simulink model "Copy_5_of_baseModel"  (R2019a)
settings: Solver=ode1  StartTime=0.0  StopTime=2.5  FixedStep=Ts_Power  RelTol=1e-3
PostLoadFcn:
  | %% Init for wind PnO models - global system parameters
  | OVERRIDE_SSN_MEMORY_LIMIT=1;
  | Ts=50e-6;
  | % Ts=50e-10;
  | Ts_Power=Ts;
  | Ts_Control=2*Ts;
  | freq = 50;
  | Fnom=freq;
  | Vac=400e3;
InitFcn:
  | %% Init for wind PnO models - global system parameters
  | OVERRIDE_SSN_MEMORY_LIMIT=1;
  | Ts=50e-6;
  | % Ts=50e-10;
  | Ts_Power=Ts;
  | Ts_Control=2*Ts;
  | freq = 50;
  | Fnom=freq;
  | Vac=225e3;
values from neighbouring files (symbols this model uses):
  ohl_posCap = (0.01e-006)*12    (= 1.2e-07)    [variable.m]
  ohl_posInd = (1.15e-3)/12    (= 9.58333333333e-05)    [variable.m]
  ohl_posR = 0.069/12    (= 0.00575)    [variable.m]
  ohl_zeroCap = (0.004e-006)*12    (= 4.8e-08)    [variable.m]
  ohl_zeroInd = (2.86e-3)/12    (= 0.000238333333333)    [variable.m]
  ohl_zeroR = 0.1725/12    (= 0.014375)    [variable.m]
  sub_posCap = sub_posCap*6    (= 9.6e-07)    [variable.m]
  sub_posInd = sub_posInd/6    (= 0.000233333333333)    [variable.m]
  sub_posR = sub_posR/6    (= 0.006)    [variable.m]
  sub_zeroCap = sub_zeroCap*6    (= 3.84e-07)    [variable.m]
  sub_zeroInd = sub_zeroInd/6    (= 0.000583333333333)    [variable.m]
  sub_zeroR = sub_zeroR/6    (= 0.015)    [variable.m]
  transfo_L1 = 0.05999374    [variable.m]
  transfo_L2 = 0.05999374    [variable.m]
  transfo_R1 = 0.000866667    [variable.m]
  transfo_R2 = 0.00086667    [variable.m]
undefined symbols (not defined in the file or in its folder): D1, D11, Delta, den, DiscIntNeverNeededParam, dx, find_system, gcbh, num, out_Buses, out_WindFarms, sps_rtmsupport
libraries: powerlib x200, simulink x96, powerlib_meascontrol x96, elements x52, eeSinusoidalMeasurement x51, simulink_extras x42, spsVIMeasurementModel x36, eePowerMeasurement x16
(part 19 of 24)

== system Copy_5_of_baseModel/SM_WT1/Overcurrent Element 2/Overcurrent Relay Scheme/Analog filtering, signal conditioning/CURRENTS ==
  Iabc : Inport
  Abs{,1..3} (4 alike) : Abs
  Add : Sum  Inputs=+++
  Complex : MagnitudeAngleToComplex
  Complex1 : MagnitudeAngleToComplex
  Complex2 : MagnitudeAngleToComplex
  Constant : Constant  Value=pi/180
  DAB - current A : Subsystem  AncestorBlock=elements/DAB  mask(Data Adquisition Board){filter=off, approx=Butterworth, order=2, numerator=[], denominator=[], freq=fCut, resdis=off, vertres=16, xmax=CurrentRange, winsize=WindowSize, G=1.0, fs=fSampling}
      mask prompts: filter "Disable Analog Filter"; approx "Filter approximation"; numerator "Free expression filter: numerator(descending order of s)"; denominator "Free expression filter: denominator:"; freq "Cut-off frequency"; resdis "Disable Vertical Resolution"; vertres "Vertical Resolution: No. of bits"; xmax "Vertical Resolution: signal range"; winsize "Window size"; G "Gain"; fs "Sampling frequency"
      mask help: Performs analog filtering, signal conditioning and sampling. A single signal is the input, a buffer with the signal samples is the output. The options include analog filter enable/disable switch, type, order and cut-off frequency of the analog filter, conditioning gain, sampling frequency, number of bits, the length of the buffer.
      mask init:
      | dab1
      mask Help: web(['file:///' which('dabdoc2.html')]);
      mask TypeOptions approx: Bessel | Tschebyscheff | Butterworth | free expression
      mask TypeOptions order: 2 | 3 | 4
      mask TypeOptions vertres: 8 | 12 | 16
      mask Display: disp('DAB')
  DAB - current B : Subsystem  AncestorBlock=elements/DAB  mask(Data Adquisition Board){filter=off, approx=Butterworth, order=2, numerator=[], denominator=[], freq=fCut, resdis=off, vertres=16, xmax=CurrentRange, winsize=WindowSize, G=1.0, fs=fSampling}
      mask prompts: filter "Disable Analog Filter"; approx "Filter approximation"; numerator "Free expression filter: numerator(descending order of s)"; denominator "Free expression filter: denominator:"; freq "Cut-off frequency"; resdis "Disable Vertical Resolution"; vertres "Vertical Resolution: No. of bits"; xmax "Vertical Resolution: signal range"; winsize "Window size"; G "Gain"; fs "Sampling frequency"
      mask help: Performs analog filtering, signal conditioning and sampling. A single signal is the input, a buffer with the signal samples is the output. The options include analog filter enable/disable switch, type, order and cut-off frequency of the analog filter, conditioning gain, sampling frequency, number of bits, the length of the buffer.
      mask init:
      | dab1
      mask Help: web(['file:///' which('dabdoc2.html')]);
      mask TypeOptions approx: Bessel | Tschebyscheff | Butterworth | free expression
      mask TypeOptions order: 2 | 3 | 4
      mask TypeOptions vertres: 8 | 12 | 16
      mask Display: disp('DAB')
  DAB - current C : Subsystem  AncestorBlock=elements/DAB  mask(Data Adquisition Board){filter=off, approx=Butterworth, order=2, numerator=[], denominator=[], freq=fCut, resdis=off, vertres=16, xmax=CurrentRange, winsize=WindowSize, G=1.0, fs=fSampling}
      mask prompts: filter "Disable Analog Filter"; approx "Filter approximation"; numerator "Free expression filter: numerator(descending order of s)"; denominator "Free expression filter: denominator:"; freq "Cut-off frequency"; resdis "Disable Vertical Resolution"; vertres "Vertical Resolution: No. of bits"; xmax "Vertical Resolution: signal range"; winsize "Window size"; G "Gain"; fs "Sampling frequency"
      mask help: Performs analog filtering, signal conditioning and sampling. A single signal is the input, a buffer with the signal samples is the output. The options include analog filter enable/disable switch, type, order and cut-off frequency of the analog filter, conditioning gain, sampling frequency, number of bits, the length of the buffer.
      mask init:
      | dab1
      mask Help: web(['file:///' which('dabdoc2.html')]);
      mask TypeOptions approx: Bessel | Tschebyscheff | Butterworth | free expression
      mask TypeOptions order: 2 | 3 | 4
      mask TypeOptions vertres: 8 | 12 | 16
      mask Display: disp('DAB')
  Demux : Demux  Outputs=3
  Gain : Gain  Gain=1/3
  Phasor IA : Subsystem  AncestorBlock=powerlib_extras/Measurements/Fourier  DialogController=POWERSYS.PowerSysDialog  mask(Fourier analyser){f1=Freq, n=1}
      mask prompts: f1 "Fundamental frequency f1 (Hz):"; n "Harmonic n (0=DC; 1=fundamental; 2=2nd harm;  ...) :"
      mask help: The Fourier block performs a Fourier analysis of the input signal over a running window of one cycle of the fundamental frequency. First and second outputs return respectively the magnitude and phase (degrees) of the harmonic component specified.
      mask init:
      | k=2-(n==0);
      | power_initmask();
      mask Help: web(psbhelp)
  Phasor IB : Subsystem  AncestorBlock=powerlib_extras/Measurements/Fourier  DialogController=POWERSYS.PowerSysDialog  mask(Fourier analyser){f1=Freq, n=1}
      mask prompts: f1 "Fundamental frequency f1 (Hz):"; n "Harmonic n (0=DC; 1=fundamental; 2=2nd harm;  ...) :"
      mask help: The Fourier block performs a Fourier analysis of the input signal over a running window of one cycle of the fundamental frequency. First and second outputs return respectively the magnitude and phase (degrees) of the harmonic component specified.
      mask init:
      | k=2-(n==0);
      | power_initmask();
      mask Help: web(psbhelp)
  Phasor IC : Subsystem  AncestorBlock=powerlib_extras/Measurements/Fourier  DialogController=POWERSYS.PowerSysDialog  mask(Fourier analyser){f1=Freq, n=1}
      mask prompts: f1 "Fundamental frequency f1 (Hz):"; n "Harmonic n (0=DC; 1=fundamental; 2=2nd harm;  ...) :"
      mask help: The Fourier block performs a Fourier analysis of the input signal over a running window of one cycle of the fundamental frequency. First and second outputs return respectively the magnitude and phase (degrees) of the harmonic component specified.
      mask init:
      | k=2-(n==0);
      | power_initmask();
      mask Help: web(psbhelp)
  Product : Product  RndMeth=Zero
  Product1 : Product  RndMeth=Zero
  Product2 : Product  RndMeth=Zero
  IAf : Outport  InitialOutput=0  VectorParamsAs1DForOutWhenUnconnected=on
  IBf : Outport  Port=2  InitialOutput=0  VectorParamsAs1DForOutWhenUnconnected=on
  ICf : Outport  Port=3  InitialOutput=0  VectorParamsAs1DForOutWhenUnconnected=on
  I0f : Outport  Port=4  InitialOutput=0  VectorParamsAs1DForOutWhenUnconnected=on
  iaf : Outport  Port=5  InitialOutput=0  VectorParamsAs1DForOutWhenUnconnected=on
  ibf : Outport  Port=6  InitialOutput=0  VectorParamsAs1DForOutWhenUnconnected=on
  icf : Outport  Port=7  InitialOutput=0  VectorParamsAs1DForOutWhenUnconnected=on
  wires:
  DAB - current C/1(d) -> icf/1, Phasor IC/1(signal)
  DAB - current B/1(d) -> ibf/1, Phasor IB/1(signal)
  DAB - current A/1(d) -> Phasor IA/1(signal), iaf/1
  Demux/2 -> DAB - current B/1(a)
  Demux/3 -> DAB - current C/1(a)
  Demux/1 -> DAB - current A/1(a)
  Iabc/1 -> Demux/1
  Phasor IA/2(angle) -> Product/1
  Constant/1 -> Product/2, Product1/2, Product2/2
  Phasor IB/2(angle) -> Product1/1
  Phasor IC/2(angle) -> Product2/1
  Phasor IA/1(magnitude) -> Complex/1
  Product/1 -> Complex/2
  Product2/1 -> Complex2/2
  Phasor IC/1(magnitude) -> Complex2/1
  Product1/1 -> Complex1/2
  Phasor IB/1(magnitude) -> Complex1/1
  Complex1/1 -> Add/2, Abs1/1
  Complex2/1 -> Add/3, Abs2/1
  Complex/1 -> Add/1, Abs/1
  Add/1 -> Gain/1
  Abs/1 -> IAf/1
  Abs1/1 -> IBf/1
  Abs2/1 -> ICf/1
  Gain/1 -> Abs3/1
  Abs3/1 -> I0f/1

== system Copy_5_of_baseModel/SM_WT1/Overcurrent Element 2/Overcurrent Relay Scheme/Phase A/Operation ==
  Iin : Inport
  " 1" : RelationalOperator  Operator=>  OutDataTypeStr=boolean  RndMeth=Nearest
  Iop : Constant  Value=Ip
  Startup : Product  RndMeth=Zero
  Step : Step  Time=0.017  SampleTime=0
  TRIP : Outport  InitialOutput=0  VectorParamsAs1DForOutWhenUnconnected=on
  wires:
  Startup/1 -> TRIP/1
  " 1"/1 -> Startup/1
  Step/1 -> Startup/2
  Iin/1 -> " 1"/1
  Iop/1 -> " 1"/2

== system Copy_5_of_baseModel/SM_WT1/Overcurrent Element 2/Overcurrent Relay Scheme/Phase B/Operation ==
  Iin : Inport
  " 1" : RelationalOperator  Operator=>  OutDataTypeStr=boolean  RndMeth=Nearest
  Iop : Constant  Value=Ip
  Startup : Product  RndMeth=Zero
  Step : Step  Time=0.017  SampleTime=0
  TRIP : Outport  InitialOutput=0  VectorParamsAs1DForOutWhenUnconnected=on
  wires:
  Iop/1 -> " 1"/2
  Iin/1 -> " 1"/1
  Step/1 -> Startup/2
  " 1"/1 -> Startup/1
  Startup/1 -> TRIP/1

== system Copy_5_of_baseModel/SM_WT1/Overcurrent Element 2/Overcurrent Relay Scheme/Phase C/Operation ==
  Iin : Inport
  " 1" : RelationalOperator  Operator=>  OutDataTypeStr=boolean  RndMeth=Nearest
  Iop : Constant  Value=Ip
  Startup : Product  RndMeth=Zero
  Step : Step  Time=0.017  SampleTime=0
  TRIP : Outport  InitialOutput=0  VectorParamsAs1DForOutWhenUnconnected=on
  wires:
  Startup/1 -> TRIP/1
  " 1"/1 -> Startup/1
  Step/1 -> Startup/2
  Iin/1 -> " 1"/1
  Iop/1 -> " 1"/2

== system Copy_5_of_baseModel/SM_WT1/Overcurrent Element 2/Overcurrent Relay Scheme/Residual/ResCurr ==
  Iin : Inport
  " 1" : RelationalOperator  Operator=>  OutDataTypeStr=boolean  RndMeth=Nearest
  Ip : Constant  Value=Iop
  Startup : Product  RndMeth=Zero
  Step : Step  Time=0.017  SampleTime=0
  TRIP : Outport  InitialOutput=0  VectorParamsAs1DForOutWhenUnconnected=on
  wires:
  Ip/1 -> " 1"/2
  Iin/1 -> " 1"/1
  Step/1 -> Startup/2
  " 1"/1 -> Startup/1
  Startup/1 -> TRIP/1

== system Copy_5_of_baseModel/SM_WT1/Overcurrent Inverse time/Overcurrent Relay Scheme/Analog filtering, signal conditioning/CURRENTS ==
  Iabc : Inport
  Abs{,1..3} (4 alike) : Abs
  Add : Sum  Inputs=+++
  Complex : MagnitudeAngleToComplex
  Complex1 : MagnitudeAngleToComplex
  Complex2 : MagnitudeAngleToComplex
  Constant : Constant  Value=pi/180
  DAB - current A : Subsystem  AncestorBlock=elements/DAB  mask(Data Adquisition Board){filter=off, approx=Butterworth, order=2, numerator=[], denominator=[], freq=fCut, resdis=off, vertres=16, xmax=CurrentRange, winsize=WindowSize, G=1.0, fs=fSampling}
      mask prompts: filter "Disable Analog Filter"; approx "Filter approximation"; numerator "Free expression filter: numerator(descending order of s)"; denominator "Free expression filter: denominator:"; freq "Cut-off frequency"; resdis "Disable Vertical Resolution"; vertres "Vertical Resolution: No. of bits"; xmax "Vertical Resolution: signal range"; winsize "Window size"; G "Gain"; fs "Sampling frequency"
      mask help: Performs analog filtering, signal conditioning and sampling. A single signal is the input, a buffer with the signal samples is the output. The options include analog filter enable/disable switch, type, order and cut-off frequency of the analog filter, conditioning gain, sampling frequency, number of bits, the length of the buffer.
      mask init:
      | dab1
      mask Help: web(['file:///' which('dabdoc2.html')]);
      mask TypeOptions approx: Bessel | Tschebyscheff | Butterworth | free expression
      mask TypeOptions order: 2 | 3 | 4
      mask TypeOptions vertres: 8 | 12 | 16
      mask Display: disp('DAB')
  DAB - current B : Subsystem  AncestorBlock=elements/DAB  mask(Data Adquisition Board){filter=off, approx=Butterworth, order=2, numerator=[], denominator=[], freq=fCut, resdis=off, vertres=16, xmax=CurrentRange, winsize=WindowSize, G=1.0, fs=fSampling}
      mask prompts: filter "Disable Analog Filter"; approx "Filter approximation"; numerator "Free expression filter: numerator(descending order of s)"; denominator "Free expression filter: denominator:"; freq "Cut-off frequency"; resdis "Disable Vertical Resolution"; vertres "Vertical Resolution: No. of bits"; xmax "Vertical Resolution: signal range"; winsize "Window size"; G "Gain"; fs "Sampling frequency"
      mask help: Performs analog filtering, signal conditioning and sampling. A single signal is the input, a buffer with the signal samples is the output. The options include analog filter enable/disable switch, type, order and cut-off frequency of the analog filter, conditioning gain, sampling frequency, number of bits, the length of the buffer.
      mask init:
      | dab1
      mask Help: web(['file:///' which('dabdoc2.html')]);
      mask TypeOptions approx: Bessel | Tschebyscheff | Butterworth | free expression
      mask TypeOptions order: 2 | 3 | 4
      mask TypeOptions vertres: 8 | 12 | 16
      mask Display: disp('DAB')
  DAB - current C : Subsystem  AncestorBlock=elements/DAB  mask(Data Adquisition Board){filter=off, approx=Butterworth, order=2, numerator=[], denominator=[], freq=fCut, resdis=off, vertres=16, xmax=CurrentRange, winsize=WindowSize, G=1.0, fs=fSampling}
      mask prompts: filter "Disable Analog Filter"; approx "Filter approximation"; numerator "Free expression filter: numerator(descending order of s)"; denominator "Free expression filter: denominator:"; freq "Cut-off frequency"; resdis "Disable Vertical Resolution"; vertres "Vertical Resolution: No. of bits"; xmax "Vertical Resolution: signal range"; winsize "Window size"; G "Gain"; fs "Sampling frequency"
      mask help: Performs analog filtering, signal conditioning and sampling. A single signal is the input, a buffer with the signal samples is the output. The options include analog filter enable/disable switch, type, order and cut-off frequency of the analog filter, conditioning gain, sampling frequency, number of bits, the length of the buffer.
      mask init:
      | dab1
      mask Help: web(['file:///' which('dabdoc2.html')]);
      mask TypeOptions approx: Bessel | Tschebyscheff | Butterworth | free expression
      mask TypeOptions order: 2 | 3 | 4
      mask TypeOptions vertres: 8 | 12 | 16
      mask Display: disp('DAB')
  Demux : Demux  Outputs=3
  Gain : Gain  Gain=1/3
  Phasor IA : Subsystem  AncestorBlock=powerlib_extras/Measurements/Fourier  DialogController=POWERSYS.PowerSysDialog  mask(Fourier analyser){f1=Freq, n=1}
      mask prompts: f1 "Fundamental frequency f1 (Hz):"; n "Harmonic n (0=DC; 1=fundamental; 2=2nd harm;  ...) :"
      mask help: The Fourier block performs a Fourier analysis of the input signal over a running window of one cycle of the fundamental frequency. First and second outputs return respectively the magnitude and phase (degrees) of the harmonic component specified.
      mask init:
      | k=2-(n==0);
      | power_initmask();
      mask Help: web(psbhelp)
  Phasor IB : Subsystem  AncestorBlock=powerlib_extras/Measurements/Fourier  DialogController=POWERSYS.PowerSysDialog  mask(Fourier analyser){f1=Freq, n=1}
      mask prompts: f1 "Fundamental frequency f1 (Hz):"; n "Harmonic n (0=DC; 1=fundamental; 2=2nd harm;  ...) :"
      mask help: The Fourier block performs a Fourier analysis of the input signal over a running window of one cycle of the fundamental frequency. First and second outputs return respectively the magnitude and phase (degrees) of the harmonic component specified.
      mask init:
      | k=2-(n==0);
      | power_initmask();
      mask Help: web(psbhelp)
  Phasor IC : Subsystem  AncestorBlock=powerlib_extras/Measurements/Fourier  DialogController=POWERSYS.PowerSysDialog  mask(Fourier analyser){f1=Freq, n=1}
      mask prompts: f1 "Fundamental frequency f1 (Hz):"; n "Harmonic n (0=DC; 1=fundamental; 2=2nd harm;  ...) :"
      mask help: The Fourier block performs a Fourier analysis of the input signal over a running window of one cycle of the fundamental frequency. First and second outputs return respectively the magnitude and phase (degrees) of the harmonic component specified.
      mask init:
      | k=2-(n==0);
      | power_initmask();
      mask Help: web(psbhelp)
  Product : Product  RndMeth=Zero
  Product1 : Product  RndMeth=Zero
  Product2 : Product  RndMeth=Zero
  IAf : Outport  InitialOutput=0  VectorParamsAs1DForOutWhenUnconnected=on
  IBf : Outport  Port=2  InitialOutput=0  VectorParamsAs1DForOutWhenUnconnected=on
  ICf : Outport  Port=3  InitialOutput=0  VectorParamsAs1DForOutWhenUnconnected=on
  I0f : Outport  Port=4  InitialOutput=0  VectorParamsAs1DForOutWhenUnconnected=on
  iaf : Outport  Port=5  InitialOutput=0  VectorParamsAs1DForOutWhenUnconnected=on
  ibf : Outport  Port=6  InitialOutput=0  VectorParamsAs1DForOutWhenUnconnected=on
  icf : Outport  Port=7  InitialOutput=0  VectorParamsAs1DForOutWhenUnconnected=on
  wires:
  DAB - current C/1(d) -> icf/1, Phasor IC/1(signal)
  DAB - current B/1(d) -> ibf/1, Phasor IB/1(signal)
  DAB - current A/1(d) -> Phasor IA/1(signal), iaf/1
  Demux/2 -> DAB - current B/1(a)
  Demux/3 -> DAB - current C/1(a)
  Demux/1 -> DAB - current A/1(a)
  Iabc/1 -> Demux/1
  Phasor IA/2(angle) -> Product/1
  Constant/1 -> Product/2, Product1/2, Product2/2
  Phasor IB/2(angle) -> Product1/1
  Phasor IC/2(angle) -> Product2/1
  Phasor IA/1(magnitude) -> Complex/1
  Product/1 -> Complex/2
  Product2/1 -> Complex2/2
  Phasor IC/1(magnitude) -> Complex2/1
  Product1/1 -> Complex1/2
  Phasor IB/1(magnitude) -> Complex1/1
  Complex1/1 -> Add/2, Abs1/1
  Complex2/1 -> Add/3, Abs2/1
  Complex/1 -> Add/1, Abs/1
  Add/1 -> Gain/1
  Abs/1 -> IAf/1
  Abs1/1 -> IBf/1
  Abs2/1 -> ICf/1
  Gain/1 -> Abs3/1
  Abs3/1 -> I0f/1

== system Copy_5_of_baseModel/SM_WT1/Overcurrent Inverse time/Overcurrent Relay Scheme/Phase A/Operation ==
  Iin : Inport
  " 1" : RelationalOperator  Operator=>  OutDataTypeStr=boolean  RndMeth=Nearest
  Iop : Constant  Value=Ip
  Startup : Product  RndMeth=Zero
  Step : Step  Time=0.017  SampleTime=0
  TRIP : Outport  InitialOutput=0  VectorParamsAs1DForOutWhenUnconnected=on
  wires:
  Startup/1 -> TRIP/1
  " 1"/1 -> Startup/1
  Step/1 -> Startup/2
  Iin/1 -> " 1"/1
  Iop/1 -> " 1"/2

== system Copy_5_of_baseModel/SM_WT1/Overcurrent Inverse time/Overcurrent Relay Scheme/Phase A/Subsystem ==
  note: Standard inverse
  note: Crtl_sig
  note: alpha
  note: Very inverse
  note: Extremely inverse
  note: Standard inverse
  note: Crtl_sig
  note: K
  note: Very inverse
  note: Extremely inverse
  "Current " : Inport
  Add1 : Sum  Inputs=+-
  Constant : Constant  Value=0.02
  Constant1 : Constant
  Constant10 : Constant  Value=0
  Constant11 : Constant
  Constant2 : Constant  Value=2
  Constant3 : Constant  Value=CtrlSig
  Constant4 : Constant  Value=0.14
  Constant5 : Constant  Value=13.5
  Constant6 : Constant  Value=80
  Constant7 : Constant  Value=CtrlSig
  Constant8 : Constant  Value=TMS
  Constant9 : Constant  Value=Iop
  Data Type Conversion : DataTypeConversion  OutDataTypeStr=double
  Divide1 : Product  Inputs=**
  Divide3 : Product  Inputs=**
  Divide4 : Product  Inputs=*/
  Divide5 : Product  Inputs=*/
  Math Function1 : Math  Operator=pow  OutputSignalType=real  SaturateOnIntegerOverflow=on
  Multiport Switch1 : MultiPortSwitch
  Multiport Switch3 : MultiPortSwitch
  Relational Operator : RelationalOperator  Operator=>  OutDataTypeStr=boolean  RndMeth=Simplest
  Time : Outport
  wires:
  Constant2/1 -> Multiport Switch3/4
  Divide4/1 -> Divide3/2
  Divide5/1 -> Math Function1/1
  Constant3/1 -> Multiport Switch3/1
  Add1/1 -> Divide4/2
  Constant11/1 -> Add1/2
  Constant9/1 -> Divide5/2
  Constant5/1 -> Multiport Switch1/3
  Multiport Switch3/1 -> Math Function1/2
  Math Function1/1 -> Add1/1
  Multiport Switch1/1 -> Divide4/1
  Constant/1 -> Multiport Switch3/2
  Constant1/1 -> Multiport Switch3/3
  Constant7/1 -> Multiport Switch1/1
  Constant6/1 -> Multiport Switch1/4
  Constant4/1 -> Multiport Switch1/2
  Constant8/1 -> Divide3/1
  "Current "/1 -> Divide5/1
  Divide3/1 -> Relational Operator/1, Divide1/1
  Constant10/1 -> Relational Operator/2
  Relational Operator/1 -> Data Type Conversion/1
  Data Type Conversion/1 -> Divide1/2
  Divide1/1 -> Time/1

== system Copy_5_of_baseModel/SM_WT1/Overcurrent Inverse time/Overcurrent Relay Scheme/Phase B/Operation ==
  Iin : Inport
  " 1" : RelationalOperator  Operator=>  OutDataTypeStr=boolean  RndMeth=Nearest
  Iop : Constant  Value=Ip
  Startup : Product  RndMeth=Zero
  Step : Step  Time=0.017  SampleTime=0
  TRIP : Outport  InitialOutput=0  VectorParamsAs1DForOutWhenUnconnected=on
  wires:
  Startup/1 -> TRIP/1
  " 1"/1 -> Startup/1
  Step/1 -> Startup/2
  Iin/1 -> " 1"/1
  Iop/1 -> " 1"/2

== system Copy_5_of_baseModel/SM_WT1/Overcurrent Inverse time/Overcurrent Relay Scheme/Phase B/Subsystem ==
  note: Standard inverse
  note: Crtl_sig
  note: alpha
  note: Very inverse
  note: Extremely inverse
  note: Standard inverse
  note: Crtl_sig
  note: K
  note: Very inverse
  note: Extremely inverse
  "Current " : Inport
  Add1 : Sum  Inputs=+-
  Constant : Constant  Value=0.02
  Constant1 : Constant
  Constant10 : Constant  Value=0
  Constant11 : Constant
  Constant2 : Constant  Value=2
  Constant3 : Constant  Value=CtrlSig
  Constant4 : Constant  Value=0.14
  Constant5 : Constant  Value=13.5
  Constant6 : Constant  Value=80
  Constant7 : Constant  Value=CtrlSig
  Constant8 : Constant  Value=TMS
  Constant9 : Constant  Value=Iop
  Data Type Conversion : DataTypeConversion  OutDataTypeStr=double
  Divide1 : Product  Inputs=**
  Divide3 : Product  Inputs=**
  Divide4 : Product  Inputs=*/
  Divide5 : Product  Inputs=*/
  Math Function1 : Math  Operator=pow  OutputSignalType=real  SaturateOnIntegerOverflow=on
  Multiport Switch1 : MultiPortSwitch
  Multiport Switch3 : MultiPortSwitch
  Relational Operator : RelationalOperator  Operator=>  OutDataTypeStr=boolean  RndMeth=Simplest
  Time : Outport
  wires:
  Constant2/1 -> Multiport Switch3/4
  Divide4/1 -> Divide3/2
  Divide5/1 -> Math Function1/1
  Constant3/1 -> Multiport Switch3/1
  Add1/1 -> Divide4/2
  Constant11/1 -> Add1/2
  Constant9/1 -> Divide5/2
  Constant5/1 -> Multiport Switch1/3
  Multiport Switch3/1 -> Math Function1/2
  Math Function1/1 -> Add1/1
  Multiport Switch1/1 -> Divide4/1
  Constant/1 -> Multiport Switch3/2
  Constant1/1 -> Multiport Switch3/3
  Constant7/1 -> Multiport Switch1/1
  Constant6/1 -> Multiport Switch1/4
  Constant4/1 -> Multiport Switch1/2
  Constant8/1 -> Divide3/1
  "Current "/1 -> Divide5/1
  Divide3/1 -> Relational Operator/1, Divide1/1
  Constant10/1 -> Relational Operator/2
  Relational Operator/1 -> Data Type Conversion/1
  Data Type Conversion/1 -> Divide1/2
  Divide1/1 -> Time/1

== system Copy_5_of_baseModel/SM_WT1/Overcurrent Inverse time/Overcurrent Relay Scheme/Phase C/Operation1 ==
  Iin : Inport
  " 1" : RelationalOperator  Operator=>  OutDataTypeStr=boolean  RndMeth=Nearest
  Iop : Constant  Value=Ip
  Startup : Product  RndMeth=Zero
  Step : Step  Time=0.017  SampleTime=0
  TRIP : Outport  InitialOutput=0  VectorParamsAs1DForOutWhenUnconnected=on
  wires:
  Startup/1 -> TRIP/1
  " 1"/1 -> Startup/1
  Step/1 -> Startup/2
  Iin/1 -> " 1"/1
  Iop/1 -> " 1"/2

== system Copy_5_of_baseModel/SM_WT1/Overcurrent Inverse time/Overcurrent Relay Scheme/Phase C/Subsystem1 ==
  note: Standard inverse
  note: Crtl_sig
  note: alpha
  note: Very inverse
  note: Extremely inverse
  note: Standard inverse
  note: Crtl_sig
  note: K
  note: Very inverse
  note: Extremely inverse
  "Current " : Inport
  Add1 : Sum  Inputs=+-
  Constant : Constant  Value=0.02
  Constant1 : Constant
  Constant10 : Constant  Value=0
  Constant11 : Constant
  Constant2 : Constant  Value=2
  Constant3 : Constant  Value=CtrlSig
  Constant4 : Constant  Value=0.14
  Constant5 : Constant  Value=13.5
  Constant6 : Constant  Value=80
  Constant7 : Constant  Value=CtrlSig
  Constant8 : Constant  Value=TMS
  Constant9 : Constant  Value=Iop
  Data Type Conversion : DataTypeConversion  OutDataTypeStr=double
  Divide1 : Product  Inputs=**
  Divide3 : Product  Inputs=**
  Divide4 : Product  Inputs=*/
  Divide5 : Product  Inputs=*/
  Math Function1 : Math  Operator=pow  OutputSignalType=real  SaturateOnIntegerOverflow=on
  Multiport Switch1 : MultiPortSwitch
  Multiport Switch3 : MultiPortSwitch
  Relational Operator : RelationalOperator  Operator=>  OutDataTypeStr=boolean  RndMeth=Simplest
  Time : Outport
  wires:
  Constant2/1 -> Multiport Switch3/4
  Divide4/1 -> Divide3/2
  Divide5/1 -> Math Function1/1
  Constant3/1 -> Multiport Switch3/1
  Add1/1 -> Divide4/2
  Constant11/1 -> Add1/2
  Constant9/1 -> Divide5/2
  Constant5/1 -> Multiport Switch1/3
  Multiport Switch3/1 -> Math Function1/2
  Math Function1/1 -> Add1/1
  Multiport Switch1/1 -> Divide4/1
  Constant/1 -> Multiport Switch3/2
  Constant1/1 -> Multiport Switch3/3
  Constant7/1 -> Multiport Switch1/1
  Constant6/1 -> Multiport Switch1/4
  Constant4/1 -> Multiport Switch1/2
  Constant8/1 -> Divide3/1
  "Current "/1 -> Divide5/1
  Divide3/1 -> Relational Operator/1, Divide1/1
  Constant10/1 -> Relational Operator/2
  Relational Operator/1 -> Data Type Conversion/1
  Data Type Conversion/1 -> Divide1/2
  Divide1/1 -> Time/1

== system Copy_5_of_baseModel/SM_WT1/Wind Type IV Detailed v2.1 - 1/Control/Measurement and Transformation/Discrete 3-phase PLL-Driven Positive-Sequence Active & Reactive Power ==
  note: Pierre Giroux, Gilbert Sybille
      | Power System Simulation Laboratory
      | IREQ, Hydro-Quebc
  note: Discrete 3-phase PLL-driven Positive-Sequence Active & Reactive Power
  Freq : Inport  PortDimensions=1
  w : Inport  Port=2  PortDimensions=1
  Vabc : Inport  Port=3  PortDimensions=3
  Iabc : Inport  Port=4  PortDimensions=3
  Deg->Rad : Gain  Gain=pi/180  SaturateOnIntegerOverflow=on  OutDataTypeStr=Inherit: Same as input  ParamDataTypeStr=Inherit: Same as input
  Discrete 3-phase PLL-Driven Positive-Sequence Fundamental Value : Subsystem  mask(Discrete 3-phase PLL-Driven Positive-Sequence Fundamental Value){Finit=Finit, Fmin=Fmin, Par_Init=Par_Vinit, Ts=Ts}
      mask prompts: Finit "Initial frequency (Hz):"; Fmin "Minimum frequency (Hz):"; Par_Init "Initial input (positive component): [ Mag  Phase-relative-to-PLL(degrees) ]"; Ts "Sample time:"
      mask help:
      | For a supplied fundamental frequency (port Freq), this discrete block computes  the positive-sequence component (Magnitude and Phase)  of a set of three balanced or unbalanced signals (port abc) which may contain harmonics.
      |  Input port "Sin_Cos" (a two-dimension signal) provides the reference frame required for the computation..
      |  First and second outputs return respectively the magnitude and phase (in degrees relative to the PLL phase)) of the fundamental.
      | For the first cycle of simulation, the outputs are held constant to the values specified by the parameter "Initial input".
      | constant to the values specified by the parameter "Initial input". The value of the parameter "Minimum frequency" is used to determine the buffer size of the "Variable Transport Delay" block found inside this subsystem.
      mask init:
      | Real_Init=Par_Init(1)*cos(pi/180*Par_Init(2));
      | Imag_Init=Par_Init(1)*sin(pi/180*Par_Init(2));
      | power_initmask();
      settings: OpenFcn=power_openblockproxy();
  Discrete 3-phase PLL-Driven Positive-Sequence Fundamental Value2 : Subsystem  mask(Discrete 3-phase PLL-Driven Positive-Sequence Fundamental Value){Finit=Finit, Fmin=Fmin, Par_Init=Par_Iinit, Ts=Ts}
      mask prompts: Finit "Initial frequency (Hz):"; Fmin "Minimum frequency (Hz):"; Par_Init "Initial input (positive component): [ Mag  Phase-relative-to-PLL(degrees) ]"; Ts "Sample time:"
      mask help:
      | For a supplied fundamental frequency (port Freq), this discrete block computes  the positive-sequence component (Magnitude and Phase)  of a set of three balanced or unbalanced signals (port abc) which may contain harmonics.
      |  Input port "Sin_Cos" (a two-dimension signal) provides the reference frame required for the computation..
      |  First and second outputs return respectively the magnitude and phase (in degrees relative to the PLL phase)) of the fundamental.
      | For the first cycle of simulation, the outputs are held constant to the values specified by the parameter "Initial input".
      | constant to the values specified by the parameter "Initial input". The value of the parameter "Minimum frequency" is used to determine the buffer size of the "Variable Transport Delay" block found inside this subsystem.
      mask init:
      | Real_Init=Par_Init(1)*cos(pi/180*Par_Init(2));
      | Imag_Init=Par_Init(1)*sin(pi/180*Par_Init(2));
      | power_initmask();
      settings: OpenFcn=power_openblockproxy();
  Gain1 : Gain  Gain=3/2  SaturateOnIntegerOverflow=on  OutDataTypeStr=Inherit: Same as input  ParamDataTypeStr=Inherit: Same as input
  Mux2 : Mux  Inputs=2
  Mux3 : Mux  Inputs=2
  Product : Product  SaturateOnIntegerOverflow=on  InputSameDT=on  OutDataTypeStr=Inherit: Same as first input
  Product1 : Product  SaturateOnIntegerOverflow=on  InputSameDT=on  OutDataTypeStr=Inherit: Same as first input
  Product2 : Product  SaturateOnIntegerOverflow=on  InputSameDT=on  OutDataTypeStr=Inherit: Same as first input
  Sum : Sum  Inputs=+-  SaturateOnIntegerOverflow=on  InputSameDT=on  OutDataTypeStr=Inherit: Same as first input
  Trigonometric Function : Trigonometry
  Trigonometric Function1 : Trigonometry  Operator=cos
  Mag_V_I : Outport  VectorParamsAs1DForOutWhenUnconnected=on
  P_Q : Outport  Port=2  VectorParamsAs1DForOutWhenUnconnected=on
  wires:
  Iabc/1 -> Discrete 3-phase PLL-Driven Positive-Sequence Fundamental Value2/3(abc)
  Discrete 3-phase PLL-Driven Positive-Sequence Fundamental Value2/1(Mag) -> Product2/2, Mux3/2
  Product2/1 -> Product1/2, Product/1
  Gain1/1 -> P_Q/1
  Mux3/1 -> Mag_V_I/1
  Product1/1 -> Mux2/2
  Product/1 -> Mux2/1
  Mux2/1 -> Gain1/1
  Trigonometric Function/1 -> Product1/1
  Trigonometric Function1/1 -> Product/2
  Deg->Rad/1 -> Trigonometric Function/1, Trigonometric Function1/1
  Sum/1 -> Deg->Rad/1
  Discrete 3-phase PLL-Driven Positive-Sequence Fundamental Value2/2(Phase) -> Sum/2
  Discrete 3-phase PLL-Driven Positive-Sequence Fundamental Value/1(Mag) -> Product2/1, Mux3/1
  Discrete 3-phase PLL-Driven Positive-Sequence Fundamental Value/2(Phase) -> Sum/1
  w/1 -> Discrete 3-phase PLL-Driven Positive-Sequence Fundamental Value2/2(w), Discrete 3-phase PLL-Driven Positive-Sequence Fundamental Value/2(w)
  Freq/1 -> Discrete 3-phase PLL-Driven Positive-Sequence Fundamental Value2/1(Freq), Discrete 3-phase PLL-Driven Positive-Sequence Fundamental Value/1(Freq)
  Vabc/1 -> Discrete 3-phase PLL-Driven Positive-Sequence Fundamental Value/3(abc)

== system Copy_5_of_baseModel/SM_WT1/Wind Type IV Detailed v2.1 - 1/Control/Measurement and Transformation/Filter ==
  Vabc_grid : Inport
  Iabc_grid_conv : Inport  Port=2
  IL : Inport  Port=3
  Vdc : Inport  Port=4
  Qref : Inport  Port=5
  Second-Order Filter{,1,4..5} (4 alike) : powerlib_meascontrol/Filters/Second-Order Filter  FilterType=Lowpass  Fo=Freq  Zeta=Zeta  Ts=Ts  Initialize=off  Vac_Init="[0,  0,  60]"  Vdc_Init=0  PlotResponse=off  FreqRange=[0, 500, 1]
      settings: SourceProductBaseCode=PS
  Second-Order Filter7 : powerlib_meascontrol/Filters/Second-Order Filter  FilterType=Lowpass  Fo=Freq  Zeta=Zeta  Ts=Ts  Initialize=on  Vac_Init=[0.8 -25 60]*0  Vdc_Init=Vdc_nom  PlotResponse=off  FreqRange=[0, 500, 1]
      settings: SourceProductBaseCode=PS
  "Vabc_grid " : Outport  VectorParamsAs1DForOutWhenUnconnected=on
  "Iabc_grid_conv " : Outport  Port=2  VectorParamsAs1DForOutWhenUnconnected=on
  "IL " : Outport  Port=3  VectorParamsAs1DForOutWhenUnconnected=on
  "Vdc " : Outport  Port=4  VectorParamsAs1DForOutWhenUnconnected=on
  "Qref " : Outport  Port=5  VectorParamsAs1DForOutWhenUnconnected=on
  wires:
  Second-Order Filter/1 -> "Vabc_grid "/1
  Second-Order Filter1/1 -> "Iabc_grid_conv "/1
  Vdc/1 -> Second-Order Filter7/1
  Second-Order Filter7/1 -> "Vdc "/1
  Qref/1 -> Second-Order Filter5/1
  Second-Order Filter5/1 -> "Qref "/1
  IL/1 -> Second-Order Filter4/1
  Second-Order Filter4/1 -> "IL "/1
  Vabc_grid/1 -> Second-Order Filter/1
  Iabc_grid_conv/1 -> Second-Order Filter1/1

== system Copy_5_of_baseModel/SM_WT1/Wind Type IV Detailed v2.1 - 2/Control/Measurement and Transformation/Discrete 3-phase PLL-Driven Positive-Sequence Active & Reactive Power ==
  note: Discrete 3-phase PLL-driven Positive-Sequence Active & Reactive Power
  note: Pierre Giroux, Gilbert Sybille
      | Power System Simulation Laboratory
      | IREQ, Hydro-Quebc
  Freq : Inport  PortDimensions=1
  w : Inport  Port=2  PortDimensions=1
  Vabc : Inport  Port=3  PortDimensions=3
  Iabc : Inport  Port=4  PortDimensions=3
  Deg->Rad : Gain  Gain=pi/180  SaturateOnIntegerOverflow=on  OutDataTypeStr=Inherit: Same as input  ParamDataTypeStr=Inherit: Same as input
  Discrete 3-phase PLL-Driven Positive-Sequence Fundamental Value : Subsystem  mask(Discrete 3-phase PLL-Driven Positive-Sequence Fundamental Value){Finit=Finit, Fmin=Fmin, Par_Init=Par_Vinit, Ts=Ts}
      mask prompts: Finit "Initial frequency (Hz):"; Fmin "Minimum frequency (Hz):"; Par_Init "Initial input (positive component): [ Mag  Phase-relative-to-PLL(degrees) ]"; Ts "Sample time:"
      mask help:
      | For a supplied fundamental frequency (port Freq), this discrete block computes  the positive-sequence component (Magnitude and Phase)  of a set of three balanced or unbalanced signals (port abc) which may contain harmonics.
      |  Input port "Sin_Cos" (a two-dimension signal) provides the reference frame required for the computation..
      |  First and second outputs return respectively the magnitude and phase (in degrees relative to the PLL phase)) of the fundamental.
      | For the first cycle of simulation, the outputs are held constant to the values specified by the parameter "Initial input".
      | constant to the values specified by the parameter "Initial input". The value of the parameter "Minimum frequency" is used to determine the buffer size of the "Variable Transport Delay" block found inside this subsystem.
      mask init:
      | Real_Init=Par_Init(1)*cos(pi/180*Par_Init(2));
      | Imag_Init=Par_Init(1)*sin(pi/180*Par_Init(2));
      | power_initmask();
      settings: OpenFcn=power_openblockproxy();
  Discrete 3-phase PLL-Driven Positive-Sequence Fundamental Value2 : Subsystem  mask(Discrete 3-phase PLL-Driven Positive-Sequence Fundamental Value){Finit=Finit, Fmin=Fmin, Par_Init=Par_Iinit, Ts=Ts}
      mask prompts: Finit "Initial frequency (Hz):"; Fmin "Minimum frequency (Hz):"; Par_Init "Initial input (positive component): [ Mag  Phase-relative-to-PLL(degrees) ]"; Ts "Sample time:"
      mask help:
      | For a supplied fundamental frequency (port Freq), this discrete block computes  the positive-sequence component (Magnitude and Phase)  of a set of three balanced or unbalanced signals (port abc) which may contain harmonics.
      |  Input port "Sin_Cos" (a two-dimension signal) provides the reference frame required for the computation..
      |  First and second outputs return respectively the magnitude and phase (in degrees relative to the PLL phase)) of the fundamental.
      | For the first cycle of simulation, the outputs are held constant to the values specified by the parameter "Initial input".
      | constant to the values specified by the parameter "Initial input". The value of the parameter "Minimum frequency" is used to determine the buffer size of the "Variable Transport Delay" block found inside this subsystem.
      mask init:
      | Real_Init=Par_Init(1)*cos(pi/180*Par_Init(2));
      | Imag_Init=Par_Init(1)*sin(pi/180*Par_Init(2));
      | power_initmask();
      settings: OpenFcn=power_openblockproxy();
  Gain1 : Gain  Gain=3/2  SaturateOnIntegerOverflow=on  OutDataTypeStr=Inherit: Same as input  ParamDataTypeStr=Inherit: Same as input
  Mux2 : Mux  Inputs=2
  Mux3 : Mux  Inputs=2
  Product : Product  SaturateOnIntegerOverflow=on  InputSameDT=on  OutDataTypeStr=Inherit: Same as first input
  Product1 : Product  SaturateOnIntegerOverflow=on  InputSameDT=on  OutDataTypeStr=Inherit: Same as first input
  Product2 : Product  SaturateOnIntegerOverflow=on  InputSameDT=on  OutDataTypeStr=Inherit: Same as first input
  Sum : Sum  Inputs=+-  SaturateOnIntegerOverflow=on  InputSameDT=on  OutDataTypeStr=Inherit: Same as first input
  Trigonometric Function : Trigonometry
  Trigonometric Function1 : Trigonometry  Operator=cos
  Mag_V_I : Outport  VectorParamsAs1DForOutWhenUnconnected=on
  P_Q : Outport  Port=2  VectorParamsAs1DForOutWhenUnconnected=on
  wires:
  Vabc/1 -> Discrete 3-phase PLL-Driven Positive-Sequence Fundamental Value/3(abc)
  Freq/1 -> Discrete 3-phase PLL-Driven Positive-Sequence Fundamental Value/1(Freq), Discrete 3-phase PLL-Driven Positive-Sequence Fundamental Value2/1(Freq)
  w/1 -> Discrete 3-phase PLL-Driven Positive-Sequence Fundamental Value/2(w), Discrete 3-phase PLL-Driven Positive-Sequence Fundamental Value2/2(w)
  Discrete 3-phase PLL-Driven Positive-Sequence Fundamental Value/2(Phase) -> Sum/1
  Discrete 3-phase PLL-Driven Positive-Sequence Fundamental Value/1(Mag) -> Mux3/1, Product2/1
  Discrete 3-phase PLL-Driven Positive-Sequence Fundamental Value2/2(Phase) -> Sum/2
  Sum/1 -> Deg->Rad/1
  Deg->Rad/1 -> Trigonometric Function1/1, Trigonometric Function/1
  Trigonometric Function1/1 -> Product/2
  Trigonometric Function/1 -> Product1/1
  Mux2/1 -> Gain1/1
  Product/1 -> Mux2/1
  Product1/1 -> Mux2/2
  Mux3/1 -> Mag_V_I/1
  Gain1/1 -> P_Q/1
  Product2/1 -> Product/1, Product1/2
  Discrete 3-phase PLL-Driven Positive-Sequence Fundamental Value2/1(Mag) -> Mux3/2, Product2/2
  Iabc/1 -> Discrete 3-phase PLL-Driven Positive-Sequence Fundamental Value2/3(abc)

== system Copy_5_of_baseModel/SM_WT1/Wind Type IV Detailed v2.1 - 2/Control/Measurement and Transformation/Filter ==
  Vabc_grid : Inport
  Iabc_grid_conv : Inport  Port=2
  IL : Inport  Port=3
  Vdc : Inport  Port=4
  Qref : Inport  Port=5
  Second-Order Filter{,1,4..5} (4 alike) : powerlib_meascontrol/Filters/Second-Order Filter  FilterType=Lowpass  Fo=Freq  Zeta=Zeta  Ts=Ts  Initialize=off  Vac_Init="[0,  0,  60]"  Vdc_Init=0  PlotResponse=off  FreqRange=[0, 500, 1]
      settings: SourceProductBaseCode=PS
  Second-Order Filter7 : powerlib_meascontrol/Filters/Second-Order Filter  FilterType=Lowpass  Fo=Freq  Zeta=Zeta  Ts=Ts  Initialize=on  Vac_Init=[0.8 -25 60]*0  Vdc_Init=Vdc_nom  PlotResponse=off  FreqRange=[0, 500, 1]
      settings: SourceProductBaseCode=PS
  "Vabc_grid " : Outport  VectorParamsAs1DForOutWhenUnconnected=on
  "Iabc_grid_conv " : Outport  Port=2  VectorParamsAs1DForOutWhenUnconnected=on
  "IL " : Outport  Port=3  VectorParamsAs1DForOutWhenUnconnected=on
  "Vdc " : Outport  Port=4  VectorParamsAs1DForOutWhenUnconnected=on
  "Qref " : Outport  Port=5  VectorParamsAs1DForOutWhenUnconnected=on
  wires:
  Iabc_grid_conv/1 -> Second-Order Filter1/1
  Vabc_grid/1 -> Second-Order Filter/1
  Second-Order Filter4/1 -> "IL "/1
  IL/1 -> Second-Order Filter4/1
  Second-Order Filter5/1 -> "Qref "/1
  Qref/1 -> Second-Order Filter5/1
  Second-Order Filter7/1 -> "Vdc "/1
  Vdc/1 -> Second-Order Filter7/1
  Second-Order Filter1/1 -> "Iabc_grid_conv "/1
  Second-Order Filter/1 -> "Vabc_grid "/1

== system Copy_5_of_baseModel/SM_WT1/Wind Type IV Detailed v2.1 - 3/Control/Measurement and Transformation/Discrete 3-phase PLL-Driven Positive-Sequence Active & Reactive Power ==
  note: Discrete 3-phase PLL-driven Positive-Sequence Active & Reactive Power
  note: Pierre Giroux, Gilbert Sybille
      | Power System Simulation Laboratory
      | IREQ, Hydro-Quebc
  Freq : Inport  PortDimensions=1
  w : Inport  Port=2  PortDimensions=1
  Vabc : Inport  Port=3  PortDimensions=3
  Iabc : Inport  Port=4  PortDimensions=3
  Deg->Rad : Gain  Gain=pi/180  SaturateOnIntegerOverflow=on  OutDataTypeStr=Inherit: Same as input  ParamDataTypeStr=Inherit: Same as input
  Discrete 3-phase PLL-Driven Positive-Sequence Fundamental Value : Subsystem  mask(Discrete 3-phase PLL-Driven Positive-Sequence Fundamental Value){Finit=Finit, Fmin=Fmin, Par_Init=Par_Vinit, Ts=Ts}
      mask prompts: Finit "Initial frequency (Hz):"; Fmin "Minimum frequency (Hz):"; Par_Init "Initial input (positive component): [ Mag  Phase-relative-to-PLL(degrees) ]"; Ts "Sample time:"
      mask help:
      | For a supplied fundamental frequency (port Freq), this discrete block computes  the positive-sequence component (Magnitude and Phase)  of a set of three balanced or unbalanced signals (port abc) which may contain harmonics.
      |  Input port "Sin_Cos" (a two-dimension signal) provides the reference frame required for the computation..
      |  First and second outputs return respectively the magnitude and phase (in degrees relative to the PLL phase)) of the fundamental.
      | For the first cycle of simulation, the outputs are held constant to the values specified by the parameter "Initial input".
      | constant to the values specified by the parameter "Initial input". The value of the parameter "Minimum frequency" is used to determine the buffer size of the "Variable Transport Delay" block found inside this subsystem.
      mask init:
      | Real_Init=Par_Init(1)*cos(pi/180*Par_Init(2));
      | Imag_Init=Par_Init(1)*sin(pi/180*Par_Init(2));
      | power_initmask();
      settings: OpenFcn=power_openblockproxy();
  Discrete 3-phase PLL-Driven Positive-Sequence Fundamental Value2 : Subsystem  mask(Discrete 3-phase PLL-Driven Positive-Sequence Fundamental Value){Finit=Finit, Fmin=Fmin, Par_Init=Par_Iinit, Ts=Ts}
      mask prompts: Finit "Initial frequency (Hz):"; Fmin "Minimum frequency (Hz):"; Par_Init "Initial input (positive component): [ Mag  Phase-relative-to-PLL(degrees) ]"; Ts "Sample time:"
      mask help:
      | For a supplied fundamental frequency (port Freq), this discrete block computes  the positive-sequence component (Magnitude and Phase)  of a set of three balanced or unbalanced signals (port abc) which may contain harmonics.
      |  Input port "Sin_Cos" (a two-dimension signal) provides the reference frame required for the computation..
      |  First and second outputs return respectively the magnitude and phase (in degrees relative to the PLL phase)) of the fundamental.
      | For the first cycle of simulation, the outputs are held constant to the values specified by the parameter "Initial input".
      | constant to the values specified by the parameter "Initial input". The value of the parameter "Minimum frequency" is used to determine the buffer size of the "Variable Transport Delay" block found inside this subsystem.
      mask init:
      | Real_Init=Par_Init(1)*cos(pi/180*Par_Init(2));
      | Imag_Init=Par_Init(1)*sin(pi/180*Par_Init(2));
      | power_initmask();
      settings: OpenFcn=power_openblockproxy();
  Gain1 : Gain  Gain=3/2  SaturateOnIntegerOverflow=on  OutDataTypeStr=Inherit: Same as input  ParamDataTypeStr=Inherit: Same as input
  Mux2 : Mux  Inputs=2
  Mux3 : Mux  Inputs=2
  Product : Product  SaturateOnIntegerOverflow=on  InputSameDT=on  OutDataTypeStr=Inherit: Same as first input
  Product1 : Product  SaturateOnIntegerOverflow=on  InputSameDT=on  OutDataTypeStr=Inherit: Same as first input
  Product2 : Product  SaturateOnIntegerOverflow=on  InputSameDT=on  OutDataTypeStr=Inherit: Same as first input
  Sum : Sum  Inputs=+-  SaturateOnIntegerOverflow=on  InputSameDT=on  OutDataTypeStr=Inherit: Same as first input
  Trigonometric Function : Trigonometry
  Trigonometric Function1 : Trigonometry  Operator=cos
  Mag_V_I : Outport  VectorParamsAs1DForOutWhenUnconnected=on
  P_Q : Outport  Port=2  VectorParamsAs1DForOutWhenUnconnected=on
  wires:
  Vabc/1 -> Discrete 3-phase PLL-Driven Positive-Sequence Fundamental Value/3(abc)
  Freq/1 -> Discrete 3-phase PLL-Driven Positive-Sequence Fundamental Value/1(Freq), Discrete 3-phase PLL-Driven Positive-Sequence Fundamental Value2/1(Freq)
  w/1 -> Discrete 3-phase PLL-Driven Positive-Sequence Fundamental Value/2(w), Discrete 3-phase PLL-Driven Positive-Sequence Fundamental Value2/2(w)
  Discrete 3-phase PLL-Driven Positive-Sequence Fundamental Value/2(Phase) -> Sum/1
  Discrete 3-phase PLL-Driven Positive-Sequence Fundamental Value/1(Mag) -> Mux3/1, Product2/1
  Discrete 3-phase PLL-Driven Positive-Sequence Fundamental Value2/2(Phase) -> Sum/2
  Sum/1 -> Deg->Rad/1
  Deg->Rad/1 -> Trigonometric Function1/1, Trigonometric Function/1
  Trigonometric Function1/1 -> Product/2
  Trigonometric Function/1 -> Product1/1
  Mux2/1 -> Gain1/1
  Product/1 -> Mux2/1
  Product1/1 -> Mux2/2
  Mux3/1 -> Mag_V_I/1
  Gain1/1 -> P_Q/1
  Product2/1 -> Product/1, Product1/2
  Discrete 3-phase PLL-Driven Positive-Sequence Fundamental Value2/1(Mag) -> Mux3/2, Product2/2
  Iabc/1 -> Discrete 3-phase PLL-Driven Positive-Sequence Fundamental Value2/3(abc)

== system Copy_5_of_baseModel/SM_WT1/Wind Type IV Detailed v2.1 - 3/Control/Measurement and Transformation/Filter ==
  Vabc_grid : Inport
  Iabc_grid_conv : Inport  Port=2
  IL : Inport  Port=3
  Vdc : Inport  Port=4
  Qref : Inport  Port=5
  Second-Order Filter{,1,4..5} (4 alike) : powerlib_meascontrol/Filters/Second-Order Filter  FilterType=Lowpass  Fo=Freq  Zeta=Zeta  Ts=Ts  Initialize=off  Vac_Init="[0,  0,  60]"  Vdc_Init=0  PlotResponse=off  FreqRange=[0, 500, 1]
      settings: SourceProductBaseCode=PS
  Second-Order Filter7 : powerlib_meascontrol/Filters/Second-Order Filter  FilterType=Lowpass  Fo=Freq  Zeta=Zeta  Ts=Ts  Initialize=on  Vac_Init=[0.8 -25 60]*0  Vdc_Init=Vdc_nom  PlotResponse=off  FreqRange=[0, 500, 1]
      settings: SourceProductBaseCode=PS
  "Vabc_grid " : Outport  VectorParamsAs1DForOutWhenUnconnected=on
  "Iabc_grid_conv " : Outport  Port=2  VectorParamsAs1DForOutWhenUnconnected=on
  "IL " : Outport  Port=3  VectorParamsAs1DForOutWhenUnconnected=on
  "Vdc " : Outport  Port=4  VectorParamsAs1DForOutWhenUnconnected=on
  "Qref " : Outport  Port=5  VectorParamsAs1DForOutWhenUnconnected=on
  wires:
  Iabc_grid_conv/1 -> Second-Order Filter1/1
  Vabc_grid/1 -> Second-Order Filter/1
  Second-Order Filter4/1 -> "IL "/1
  IL/1 -> Second-Order Filter4/1
  Second-Order Filter5/1 -> "Qref "/1
  Qref/1 -> Second-Order Filter5/1
  Second-Order Filter7/1 -> "Vdc "/1
  Vdc/1 -> Second-Order Filter7/1
  Second-Order Filter1/1 -> "Iabc_grid_conv "/1
  Second-Order Filter/1 -> "Vabc_grid "/1
